simulink model "SBR_NonLinear"  (R2025b)
settings: Solver=VariableStepAuto  StartTime=0.0  StopTime=4  FixedStep=1e-6  RelTol=1e-9
values from neighbouring files (symbols this model uses):
  b_body = 10e-3    (= 0.01)    [SBR_NonLinear_Data.m]
  g = 9.81    [SBR_NonLinear_Data.m]
  h_body = 20e-3    (= 0.02)    [SBR_NonLinear_Data.m]
  J_body = 1/12*m_body*h_body^2    (= 6.66666666667e-06)    [SBR_NonLinear_Data.m]
  Jw = (0.5 * m_w * r_w^2) + (1/12 * m_w * h_w^2)    (= 5.96107666667e-05)    [SBR_NonLinear_Data.m]
  k_eff = 0.8    [SBR_NonLinear_Data.m]
  k_gear = 120    [SBR_NonLinear_Data.m]
  KePhi = 0.336    [SBR_NonLinear_Data.m]
  La = 50e-6    (= 5e-05)    [SBR_NonLinear_Data.m]
  m_body = 200e-3    (= 0.2)    [SBR_NonLinear_Data.m]
  mu_w = 0.2    [SBR_NonLinear_Data.m]
  powerConv_kp = 6/Vdd    (= 1.81818181818)    [SBR_NonLinear_Data.m]
  Q_pwm = Vdd/(2^n_pwm)    (= 0.012890625)    [SBR_NonLinear_Data.m]
  r_w = 77.1e-3    (= 0.0771)    [SBR_NonLinear_Data.m]
  Ra = 3.5    [SBR_NonLinear_Data.m]
  Vdd = 3.3    [SBR_NonLinear_Data.m]
undefined symbols (not defined in the file or in its folder): l, m
libraries: simulink x2, slpidlib x1
settings Model: Creator=banom  LastModifiedBy=spera

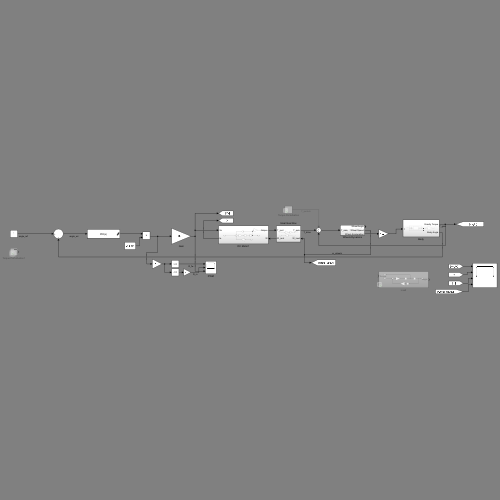
[thumbnail: Simulink's stored preview of the top-level diagram]
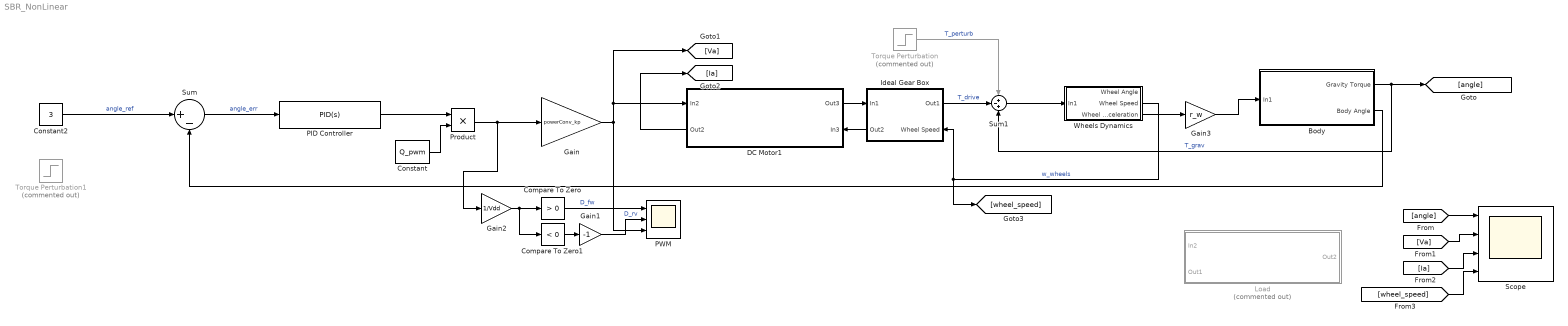
== system SBR_NonLinear ==
  Body : Subsystem
  Compare To Zero : simulink/Logic and Bit Operations/Compare To Zero  relop=>  OutDataTypeStr=boolean
  Compare To Zero1 : simulink/Logic and Bit Operations/Compare To Zero  relop=<  OutDataTypeStr=boolean
  Constant : Constant  Value=Q_pwm
  Constant2 : Constant  Value=3
  DC Motor1 : Subsystem
      settings: PortSchema="{\"entries\":[{\"content\":{\"sides\":[{\"content\":{\"connectorIds\":[\"In1\",\"Out2\"]},\"type\":\"ConnectorPlacement.EquallySpacedRectSide\",\"uuid\":\"1f0826b0-c8fa-4dfd-b84b-9705fcde42a6\"},{\"content\":{\"connectorIds\":[\"Out1\",\"In2\"],\"side\":\"RIGHT\"},\"type\":\"ConnectorPlacement.EquallySpacedRectSide\",\"uuid\":\"1ff7b257-b76c-4c51-8a66-4278f6333452\"},{\"content\":{\"side\":\"TOP\"},\"type\":\"ConnectorPlacement.EquallySpacedRectSide\",\"uuid\":\"88c49e0f-3c27-4744-b6e4-e81bc6360818\"},{\"content\":{\"side\":\"BOTTOM\"},\"type\":\"ConnectorPlacement.EquallySpacedRectSide\",\"uuid\":\"43e2c16a-78aa-43f1-b412-49aa61b6e3d2\"}]},\"type\":\"ConnectorPlacement.EquallySpacedConnector\",\"uuid\":\"80e29701-d3dc-4e72-874c-b1f53b63a851\"}],\"packageUris\":[\"http://schema.mathworks.com/mf0/Connector/R2020b\"],\"version\":\"1.0\"}"
  Gain : Gain  Gain=powerConv_kp
  Gain1 : Gain  Gain=-1
  Gain2 : Gain  Gain=1/Vdd
  Gain3 : Gain  Gain=r_w
  Ideal Gear Box : Subsystem
      settings: PortSchema="{\"entries\":[{\"content\":{\"sides\":[{\"content\":{\"connectorIds\":[\"Out2\",\"In1\"]},\"type\":\"ConnectorPlacement.EquallySpacedRectSide\",\"uuid\":\"1f0826b0-c8fa-4dfd-b84b-9705fcde42a6\"},{\"content\":{\"connectorIds\":[\"In2\",\"Out1\"],\"side\":\"RIGHT\"},\"type\":\"ConnectorPlacement.EquallySpacedRectSide\",\"uuid\":\"1ff7b257-b76c-4c51-8a66-4278f6333452\"},{\"content\":{\"side\":\"TOP\"},\"type\":\"ConnectorPlacement.EquallySpacedRectSide\",\"uuid\":\"88c49e0f-3c27-4744-b6e4-e81bc6360818\"}]},\"type\":\"ConnectorPlacement.EquallySpacedConnector\",\"uuid\":\"80e29701-d3dc-4e72-874c-b1f53b63a851\"}],\"packageUris\":[\"http://schema.mathworks.com/mf0/Connector/R2020b\"],\"version\":\"1.0\"}"
  Load : Subsystem  Commented=on
      settings: PortSchema="{\"entries\":[{\"content\":{\"sides\":[{\"content\":{\"connectorIds\":[\"In1\",\"Out2\"]},\"type\":\"ConnectorPlacement.EquallySpacedRectSide\",\"uuid\":\"1c09c499-258b-46cd-a8f7-6b056a17df42\"},{\"content\":{\"connectorIds\":[\"Out1\"],\"side\":\"RIGHT\"},\"type\":\"ConnectorPlacement.EquallySpacedRectSide\",\"uuid\":\"0cb6394e-ddf7-4c56-ac30-e644da1ce5fd\"},{\"content\":{\"side\":\"TOP\"},\"type\":\"ConnectorPlacement.EquallySpacedRectSide\",\"uuid\":\"dcbd258b-94e7-48e5-b6b7-c73ca781daf7\"}]},\"type\":\"ConnectorPlacement.EquallySpacedConnector\",\"uuid\":\"f73fe1be-6e66-458f-83d9-ff51acf193bd\"}],\"packageUris\":[\"http://schema.mathworks.com/mf0/Connector/R2020b\"],\"version\":\"1.0\"}"
  PID Controller : slpidlib/PID Controller  Controller=PID  Form=Parallel  TimeDomain=Continuous-time  UseExternalTs=off  SampleTime=-1  IntegratorMethod=Forward Euler  FilterMethod=Forward Euler  ControllerParametersSource=internal  P=10  I=0.02  UseKiTs=off  D=0.04  UseExternalDerivativeSource=off  N=100  UseFilter=on  TunerSelectOption=Transfer Function Based (PID Tuner App)  InitialConditionSource=internal  InitialConditionForIntegrator=0  InitialConditionForFilter=0  DifferentiatorICPrevScaledInput=0  ExternalReset=none  TrackingMode=off  Kt=1  LimitOutput=on  SatLimitsSource=internal  UpperSaturationLimit=255  LowerSaturationLimit=-255  LinearizeAsGain=on  AntiWindupMode=none  Kb=1  LimitIntegrator=off  UpperIntegratorSaturationLimit=inf  LowerIntegratorSaturationLimit=-inf  POutMin=[]  POutMax=[]  IOutMin=[]  IOutMax=[]  DOutMin=[]  DOutMax=[]  NOutMin=[]  NOutMax=[]  SumOutMin=[]  SumOutMax=[]  SaturationOutMin=[]  SaturationOutMax=[]  PParamMin=[]  PParamMax=[]  IParamMin=[]  IParamMax=[]  DParamMin=[]  DParamMax=[]  NParamMin=[]  NParamMax=[]  KbParamMin=[]  KbParamMax=[]  KtParamMin=[]  KtParamMax=[]  KbOutMin=[]  KbOutMax=[]  KtOutMin=[]  KtOutMax=[]  IntegratorOutMin=[]  IntegratorOutMax=[]  FilterOutMin=[]  FilterOutMax=[]  SumI1OutMin=[]  SumI1OutMax=[]  SumI2OutMin=[]  SumI2OutMax=[]  SumI3OutMin=[]  SumI3OutMax=[]  SumI4OutMin=[]  SumI4OutMax=[]  SumDOutMin=[]  SumDOutMax=[]  DifferentiatorOutMin=[]  DifferentiatorOutMax=[]  FilterDiffOutCoefMin=[]  FilterDiffOutCoefMax=[]  ReciprocalOutMin=[]  ReciprocalOutMax=[]  SumDenOutMin=[]  SumDenOutMax=[]  SumNumOutMin=[]  SumNumOutMax=[]  DivideOutMin=[]  DivideOutMax=[]  UdiffTsProdOutMin=[]  UdiffTsProdOutMax=[]  NTsProdOutMin=[]  NTsProdOutMax=[]  UintegralTsProdOutMin=[]  UintegralTsProdOutMax=[]  UngainTsProdOutMin=[]  UngainTsProdOutMax=[]  ClampingZeroOutDataTypeStr=Inherit: Inherit via back propagation  ClampingZeroOutMin=[]  ClampingZeroOutMax=[]  FilterDenConstantOutDataTypeStr=Inherit: Inherit via back propagation  FilterDenConstantOutMin=[]  FilterDenConstantOutMax=[]  PCopyOutDataTypeStr=Inherit: Inherit via back propagation  PCopyOutMin=[]  PCopyOutMax=[]  NCopyOutDataTypeStr=Inherit: Inherit via back propagation  NCopyOutMin=[]  NCopyOutMax=[]  IntegratorContinuousStateAttributes=''  IntegratorStateMustResolveToSignalObject=off  IntegratorRTWStateStorageClass=Auto  FilterContinuousStateAttributes=''  FilterStateMustResolveToSignalObject=off  FilterRTWStateStorageClass=Auto  ParallelPVariant=InternalParameters  IdealPVariant=Disabled  IVariant=InternalParameters  DVariant=InternalParameters  IntegratorVariant=Continuous  SatVariant=Enabled  AWVariant=Passthrough  PCopyVariant=Disabled  TRVariant=Disabled  FdbkBlocksVariant=Forward  IdealPFdbkVariant=Disabled  SatFdbkVariant=Disabled  DerivativeFilterVariant=ContFilter  NVariant=InternalParameters  NCopyVariant=Disabled  FilterICVariant=InternalICsFilter  IntegratorICVariant=InternalICs  ExternalResetVariant=Disabled  TRSumVariant=Passthrough  SumFdbkVariant=Disabled  SumVariant=Sum_PID  TsampFilterVariant=InternalTs  TsampNgainVariant=Passthrough  TsampIntegralVariant=Disabled_SignalSpec  ExternalSaturationOutDataTypeStr=Inherit: Same as second input  DerivativeSourceVariant=ErrorSignal  PreIntVariant=InternalPreInt
  PWM : Scope  NumInputPorts=3
      settings: ActiveDisplayYMinimum=-0.12499999999999997  ActiveDisplayYMaximum=1.125  DataLoggingVariableName=ScopeData3
  Product : Product
  Scope : Scope  NumInputPorts=4
      settings: ActiveDisplayYMinimum=-0.049049998960034709  ActiveDisplayYMaximum=0.049049999879650211
  Sum : Sum  Inputs=|+-
  Sum1 : Sum  Inputs=+-+
  Torque Perturbation : Step  Commented=on  SampleTime=0
  Torque Perturbation1 : Step  Commented=on  SampleTime=0
  Wheels Dynamics : Subsystem
  wires:
  Gain/1 -> PWM/3, DC Motor1/1(In2), [Va]
  PID Controller/1 -> Product/1
  Constant/1 -> Product/2
  Compare To Zero1/1 -> Gain1/1
  Compare To Zero/1 -> PWM/1  "D_fw"
  Gain1/1 -> PWM/2  "D_rv"
  Product/1 -> Gain2/1, Gain/1
  DC Motor1/1(Out3) -> Ideal Gear Box/2(In1)
  Sum1/1 -> Wheels Dynamics/1(In1)
  Ideal Gear Box/2(Out1) -> Sum1/2  "T_drive"
  Body/1(Gravity Torque) -> Sum1/3, [angle]  "T_grav"
  Torque Perturbation/1 -> Sum1/1  "T_perturb"
  Wheels Dynamics/2(Wheel Speed) -> [wheel_speed], Ideal Gear Box/1(Wheel Speed)  "w_wheels"
  Sum/1 -> PID Controller/1  "angle_err"
  Gain2/1 -> Compare To Zero1/1, Compare To Zero/1
  Wheels Dynamics/3(Wheel Acceleration) -> Gain3/1
  Gain3/1 -> Body/1(In1)
  [angle] -> Scope/1
  DC Motor1/2(Out2) -> [Ia]
  [Va] -> Scope/2
  [Ia] -> Scope/3
  [wheel_speed] -> Scope/4
  Ideal Gear Box/1(Out2) -> DC Motor1/2(In3)
  Body/2(Body Angle) -> Sum/2
  Constant2/1 -> Sum/1  "angle_ref"

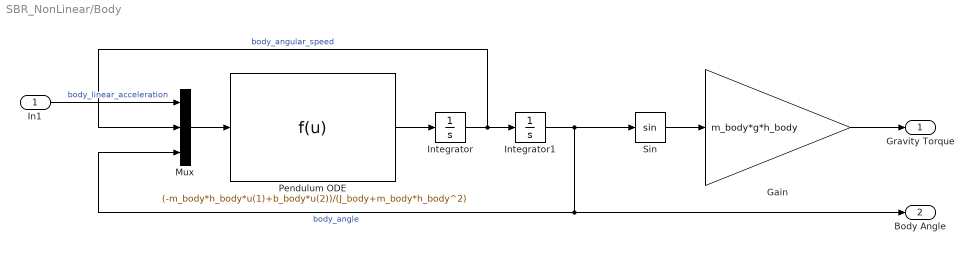
== system SBR_NonLinear/Body ==
  In1 : Inport
  Gain : Gain  Gain=m_body*g*h_body
  Integrator : Integrator  LimitOutput=on  UpperSaturationLimit=100  LowerSaturationLimit=-100
  Integrator1 : Integrator  LimitOutput=on  UpperSaturationLimit=90  LowerSaturationLimit=-90
  Mux : Mux  Inputs=3
  Pendulum ODE : Fcn  Expr=(-m_body*h_body*u(1)+b_body*u(2))/(J_body+m_body*h_body^2)
  Sin : Trigonometry
  Gravity Torque : Outport
  Body Angle : Outport  Port=2
  wires:
  Sin/1 -> Gain/1
  Gain/1 -> Gravity Torque/1
  Mux/1 -> Pendulum ODE/1
  In1/1 -> Mux/1  "body_linear_acceleration"
  Pendulum ODE/1 -> Integrator/1
  Integrator/1 -> Mux/2, Integrator1/1  "body_angular_speed"
  Integrator1/1 -> Mux/3, Body Angle/1, Sin/1  "body_angle"

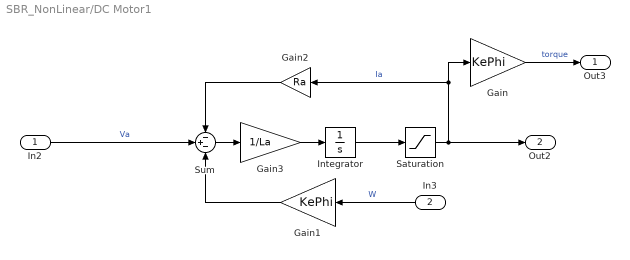
== system SBR_NonLinear/DC Motor1 ==
  In2 : Inport
  In3 : Inport  Port=2
  Gain : Gain  Gain=KePhi
  Gain1 : Gain  Gain=KePhi
  Gain2 : Gain  Gain=Ra
  Gain3 : Gain  Gain=1/La
  Integrator : Integrator
  Saturation : Saturate  UpperLimit=2  LowerLimit=-2
  Sum : Sum  Inputs=-+-
  Out3 : Outport
  Out2 : Outport  Port=2
  wires:
  In3/1 -> Gain1/1  "W"
  Gain/1 -> Out3/1  "torque"
  Gain3/1 -> Integrator/1
  Saturation/1 -> Gain2/1, Gain/1, Out2/1  "Ia"
  Gain1/1 -> Sum/3
  In2/1 -> Sum/2  "Va"
  Gain2/1 -> Sum/1
  Sum/1 -> Gain3/1
  Integrator/1 -> Saturation/1

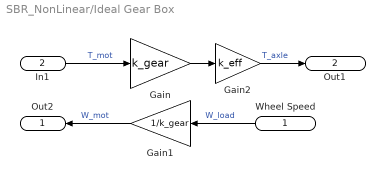
== system SBR_NonLinear/Ideal Gear Box ==
  Wheel Speed : Inport
  In1 : Inport  Port=2
  Gain : Gain  Gain=k_gear
  Gain1 : Gain  Gain=1/k_gear
  Gain2 : Gain  Gain=k_eff
  Out2 : Outport
  Out1 : Outport  Port=2
  wires:
  In1/1 -> Gain/1  "T_mot"
  Gain1/1 -> Out2/1  "W_mot"
  Wheel Speed/1 -> Gain1/1  "W_load"
  Gain/1 -> Gain2/1
  Gain2/1 -> Out1/1  "T_axle"

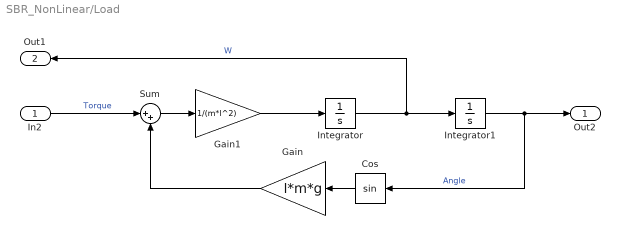
== system SBR_NonLinear/Load ==
  In2 : Inport
  Cos : Trigonometry
  Gain : Gain  Gain=l*m*g
  Gain1 : Gain  Gain=1/(m*l^2)
  Integrator : Integrator
  Integrator1 : Integrator
  Sum : Sum  Inputs=|++
  Out2 : Outport
  Out1 : Outport  Port=2
  wires:
  In2/1 -> Sum/1  "Torque"
  Cos/1 -> Gain/1
  Gain/1 -> Sum/2
  Integrator1/1 -> Cos/1, Out2/1  "Angle"
  Integrator/1 -> Out1/1, Integrator1/1  "W"
  Sum/1 -> Gain1/1
  Gain1/1 -> Integrator/1

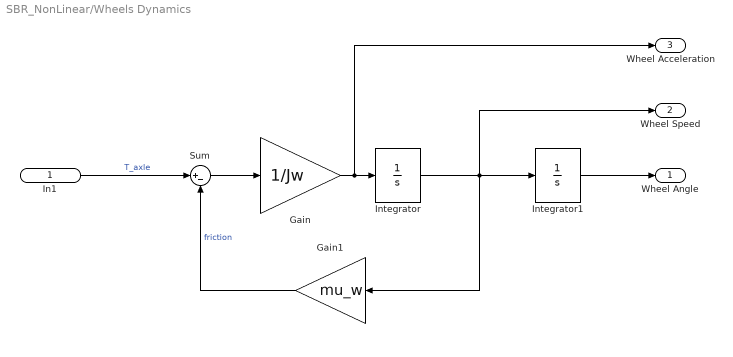
== system SBR_NonLinear/Wheels Dynamics ==
  In1 : Inport
  Gain : Gain  Gain=1/Jw
  Gain1 : Gain  Gain=mu_w
  Integrator : Integrator  LimitOutput=on  UpperSaturationLimit=100  LowerSaturationLimit=-100
  Integrator1 : Integrator
  Sum : Sum  Inputs=|+-
  Wheel Angle : Outport
  Wheel Speed : Outport  Port=2
  Wheel Acceleration : Outport  Port=3
  wires:
  In1/1 -> Sum/1  "T_axle"
  Gain1/1 -> Sum/2  "friction"
  Sum/1 -> Gain/1
  Gain/1 -> Wheel Acceleration/1, Integrator/1
  Integrator/1 -> Gain1/1, Wheel Speed/1, Integrator1/1
  Integrator1/1 -> Wheel Angle/1
